simulink library "demo_lib_ctl"  (R2024a)
settings: Solver=VariableStepAuto  StartTime=0.0  StopTime=10.0  RelTol=1e-3
undefined symbols (not defined in the file or in its folder): Controller1_data, Controller1_DT, Controller1_LT, Controller1_params, Controller1_PT, Controller2_data, Controller2_DT, Controller2_LT, Controller2_params, Controller2_PT, extrinsic
settings Model: Creator=luka  LastModifiedBy=luka

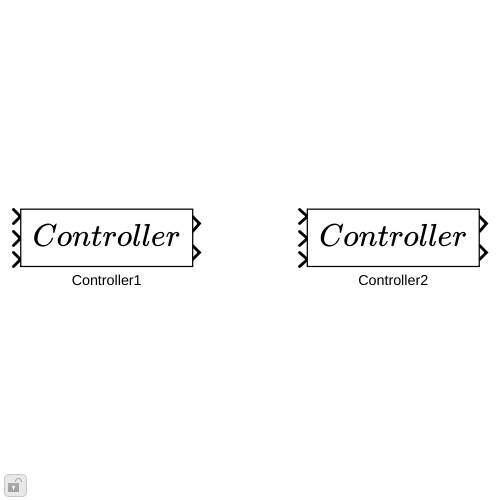
[thumbnail: Simulink's stored preview of the top-level diagram]
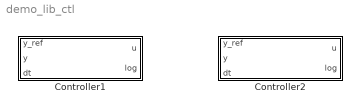
== system demo_lib_ctl ==
  Controller1 : Subsystem  Tag=__cs_m_ctl;  mask{iid__=[0], pid__=[67 111 110 116 114 111 108 108 101 114 49 58 100 101 109 111 95 108 105 98], LogEntryType=Controller1_LT, params=Controller1_params, data=Controller1_data, ParamsType=Controller1_PT, DataType=Controller1_DT, u_ic=0}
      mask prompts: params "Parameter struct:"
  Controller2 : Subsystem  Tag=__cs_py_ctl;  mask{iid__=[0], pid__=[67 111 110 116 114 111 108 108 101 114 50 58 100 101 109 111 95 108 105 98], LogEntryType=Controller2_LT, params=Controller2_params, data=Controller2_data, ParamsType=Controller2_PT, DataType=Controller2_DT, u_ic=0}
      mask prompts: params "Parameter struct:"

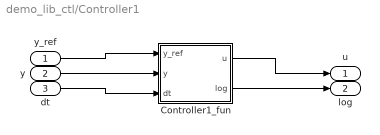
== system demo_lib_ctl/Controller1 ==
  y_ref : Inport
  y : Inport  Port=2
  dt : Inport  Port=3
  Controller1_fun : MATLAB Function  TreatAsAtomicUnit=on
  u : Outport
  log : Outport  Port=2
  wires:
  y_ref/1 -> Controller1_fun/1(y_ref)
  y/1 -> Controller1_fun/2(y)
  dt/1 -> Controller1_fun/3(dt)
  Controller1_fun/1(u) -> u/1
  Controller1_fun/2(log) -> log/1

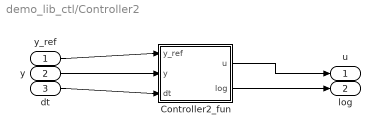
== system demo_lib_ctl/Controller2 ==
  y_ref : Inport
  y : Inport  Port=2
  dt : Inport  Port=3
  Controller2_fun : MATLAB Function  TreatAsAtomicUnit=on
  u : Outport
  log : Outport  Port=2
  wires:
  y_ref/1 -> Controller2_fun/1(y_ref)
  y/1 -> Controller2_fun/2(y)
  dt/1 -> Controller2_fun/3(dt)
  Controller2_fun/1(u) -> u/1
  Controller2_fun/2(log) -> log/1

== matlab function demo_lib_ctl/Controller2/Controller2_fun ==
  settings: updateMethod=DISCRETE
  data: y_ref input; u output; y input; dt input; log output LogEntryType; iid__ parameter uint8; pid__ parameter uint8; data parameter DataType; params parameter ParamsType; u_ic parameter double
% __classname:="Controller2";
% __lib_name:="demo_lib";
% __comp_type:="ctl";
% __plugin_type:="py";
% __fnname:="fcn_80eded98d5f341538a38bb328561e47a";
% __input_args:="y_ref, y, dt, u_ic, params, data, pid__, iid__";
% __output_args:=" u";
% __ctor_args:="'Params', params, 'Data', data, 'pid', pid__, 'iid', iid__";
% __cfg_args:="u_ic, size(y), size(y_ref)";
% __step_args:="y_ref, y, dt";
function [  u, log] = fcn(y_ref, y, dt, iid__, pid__, data, params, u_ic)
    coder.extrinsic('fcn_80eded98d5f341538a38bb328561e47a_ext');
u = u_ic;
data_n = data;
;
        [data_n,  u] = fcn_80eded98d5f341538a38bb328561e47a_ext(y_ref, y, dt, u_ic, params, data, pid__, iid__);
        log = eval_log(data_n);
end

function log = eval_log(data)
        log.d3 = data.d3;

end

== matlab function demo_lib_ctl/Controller1/Controller1_fun ==
  settings: updateMethod=DISCRETE
  data: y_ref input; u output; y input; dt input; log output LogEntryType; extrinsic parameter int32; iid__ parameter uint8; pid__ parameter uint8; data parameter DataType; params parameter ParamsType; u_ic parameter double
% __classname:="Controller1";
% __lib_name:="demo_lib";
% __comp_type:="ctl";
% __plugin_type:="mat";
% __fnname:="fcn_5993e002d666431f8166716e2a8f65b9";
% __input_args:="y_ref, y, dt, u_ic, params, data, pid__, iid__";
% __output_args:=" u";
% __ctor_args:="'Params', params, 'Data', data, 'pid', pid__, 'iid', iid__";
% __cfg_args:="u_ic, size(y), size(y_ref)";
% __step_args:="y_ref, y, dt";
function [  u, log] = fcn(y_ref, y, dt, extrinsic, iid__, pid__, data, params, u_ic)
    coder.extrinsic('fcn_5993e002d666431f8166716e2a8f65b9_ext');
    if extrinsic
u = u_ic;;
        [  u, log] = fcn_5993e002d666431f8166716e2a8f65b9_ext(y_ref, y, dt, u_ic, params, data, pid__, iid__);
    else
        [  u, log] = fcn_5993e002d666431f8166716e2a8f65b9(y_ref, y, dt, u_ic, params, data, pid__, iid__);
    end 
end

 
function [  u, log] = fcn_5993e002d666431f8166716e2a8f65b9(y_ref, y, dt, u_ic, params, data, pid__, iid__)
    persistent obj
    if isempty(obj)
        obj = Controller1('Params', params, 'Data', data, 'pid', pid__, 'iid', iid__);
        obj = obj.configure(u_ic, size(y), size(y_ref));
    end
    [obj,  u] = obj.step(y_ref, y, dt);
    log = eval_log(obj.data);
end

function log = eval_log(data)
        log.log1 = data.log1;

end
